simulink model "QCS_Closed_Loop_Sim"  (Simulink 9.1)
settings: Solver=FixedStepAuto  StartTime=0.0  StopTime=3  FixedStep=Ts  RelTol=1e-3  EnableMultiTasking=on
libraries: cstblocks x13
settings Model: SuppressorTable=22 serialization::archive 11 0 6 0 0 0 0 0  Creator=Mokrane  LastModifiedBy=Mokrane
settings DataIOCC: LimitDataPoints=on  SignalLoggingSaveFormat=ModelDataLogs  SignalLoggingName=sigsOut
settings OptimizationCC: LifeSpan=auto
settings DebuggingCC: SaveWithParameterizedLinksMsg=none  SignalResolutionControl=TryResolveAllWithWarning  MultiTaskDSMMsg=warning  MultiTaskCondExecSysMsg=none  SFUnexpectedBacktrackingDiag=error  SFNoUnconditionalDefaultTransitionDiag=error  SFExecutionAtInitializationDiag=warning
settings HardwareCC: TargetUnknown=on
settings CodeAppCC: StateflowObjectComments=off

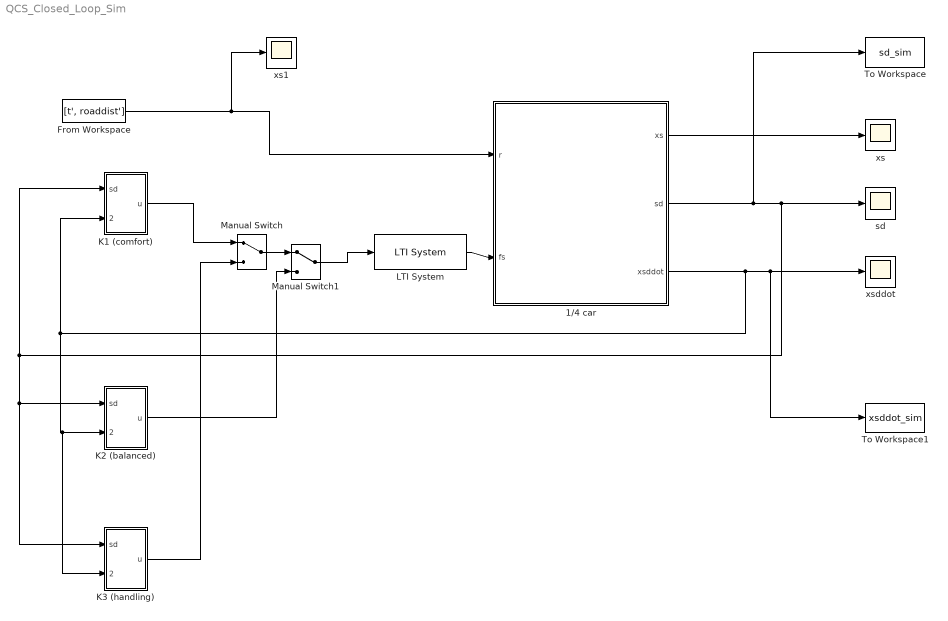
== system QCS_Closed_Loop_Sim ==
  1/4 car : Subsystem
  From Workspace : FromWorkspace  VariableName=[t', roaddist']  SampleTime=0
  K1 (comfort) : Subsystem
  K2 (balanced) : Subsystem
  K3 (handling) : Subsystem
  LTI System : cstblocks/LTI System  sys=Act  IC=[]
  Manual Switch : ManualSwitch
  Manual Switch1 : ManualSwitch
  To Workspace : ToWorkspace  VariableName=sd_sim  SaveFormat=Timeseries  SampleTime=-1
  To Workspace1 : ToWorkspace  VariableName=xsddot_sim  SaveFormat=Timeseries  SampleTime=-1
  sd : Scope
  xs : Scope
  xs1 : Scope
  xsddot : Scope
  wires:
  From Workspace/1 -> xs1/1, 1/4 car/1(r)
  1/4 car/1(xs) -> xs/1
  1/4 car/3(xsddot) -> K3 (handling)/2(xsddot), K2 (balanced)/2(xsddot), K1 (comfort)/2(xsddot), To Workspace1/1, xsddot/1
  1/4 car/2(sd) -> To Workspace/1, K3 (handling)/1(sd), K2 (balanced)/1(sd), K1 (comfort)/1(sd), sd/1
  LTI System/1 -> 1/4 car/2(fs)
  K3 (handling)/1(u) -> Manual Switch/2
  Manual Switch/1 -> Manual Switch1/1
  K1 (comfort)/1(u) -> Manual Switch/1
  K2 (balanced)/1(u) -> Manual Switch1/2
  Manual Switch1/1 -> LTI System/1

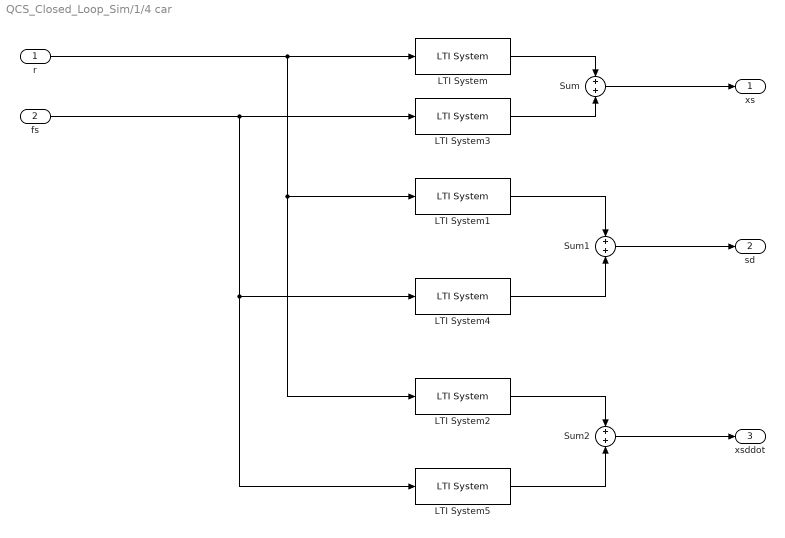
== system QCS_Closed_Loop_Sim/1/4 car ==
  r : Inport
  fs : Inport  Port=2
  LTI System : cstblocks/LTI System  sys=G11  IC=[]
  LTI System1 : cstblocks/LTI System  sys=G21  IC=[]
  LTI System2 : cstblocks/LTI System  sys=G31  IC=[]
  LTI System3 : cstblocks/LTI System  sys=G12  IC=[]
  LTI System4 : cstblocks/LTI System  sys=G22  IC=[]
  LTI System5 : cstblocks/LTI System  sys=G32  IC=[]
  Sum : Sum
  Sum1 : Sum
  Sum2 : Sum
  xs : Outport
  sd : Outport  Port=2
  xsddot : Outport  Port=3
  wires:
  Sum2/1 -> xsddot/1
  Sum/1 -> xs/1
  LTI System5/1 -> Sum2/2
  LTI System4/1 -> Sum1/2
  r/1 -> LTI System2/1, LTI System1/1, LTI System/1
  LTI System1/1 -> Sum1/1
  fs/1 -> LTI System5/1, LTI System4/1, LTI System3/1
  Sum1/1 -> sd/1
  LTI System2/1 -> Sum2/1
  LTI System3/1 -> Sum/2
  LTI System/1 -> Sum/1

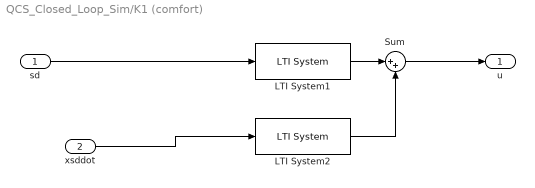
== system QCS_Closed_Loop_Sim/K1 (comfort) ==
  sd : Inport
  xsddot : Inport  Port=2
  LTI System1 : cstblocks/LTI System  sys=K1_1  IC=[]
  LTI System2 : cstblocks/LTI System  sys=K1_2  IC=[]
  Sum : Sum  Inputs=|++
  u : Outport
  wires:
  LTI System2/1 -> Sum/2
  xsddot/1 -> LTI System2/1
  sd/1 -> LTI System1/1
  Sum/1 -> u/1
  LTI System1/1 -> Sum/1

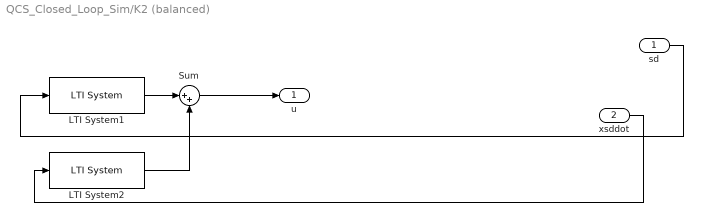
== system QCS_Closed_Loop_Sim/K2 (balanced) ==
  sd : Inport
  xsddot : Inport  Port=2
  LTI System1 : cstblocks/LTI System  sys=K2_1  IC=[]
  LTI System2 : cstblocks/LTI System  sys=K2_2  IC=[]
  Sum : Sum  Inputs=|++
  u : Outport
  wires:
  LTI System2/1 -> Sum/2
  xsddot/1 -> LTI System2/1
  sd/1 -> LTI System1/1
  Sum/1 -> u/1
  LTI System1/1 -> Sum/1

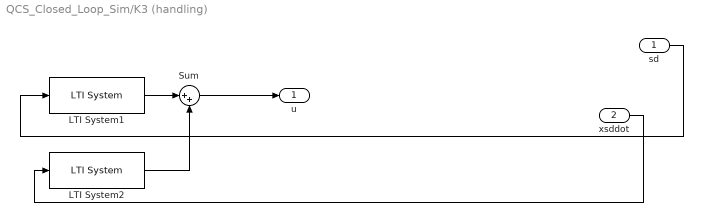
== system QCS_Closed_Loop_Sim/K3 (handling) ==
  sd : Inport
  xsddot : Inport  Port=2
  LTI System1 : cstblocks/LTI System  sys=K3_1  IC=[]
  LTI System2 : cstblocks/LTI System  sys=K3_2  IC=[]
  Sum : Sum  Inputs=|++
  u : Outport
  wires:
  LTI System2/1 -> Sum/2
  xsddot/1 -> LTI System2/1
  sd/1 -> LTI System1/1
  Sum/1 -> u/1
  LTI System1/1 -> Sum/1
